simulink model "TST_SATELLITE_A_FAIRE"  (Simulink 8.2)
settings: Solver=ode45  StartTime=0.0  StopTime=60  RelTol=1e-3
values from neighbouring files (symbols this model uses):
  qsc_I_ini = [0 0 0 1]'    [iniSATELLITE.m]
  RW1axe_B = [1 0 0]'    [iniSATELLITE.m]
  RW1inertie_inv = 1/RW1inertie    (= 2439.02439024)    [iniSATELLITE.m]
  RW2axe_B = [0 1 0]'    [iniSATELLITE.m]
  RW2inertie_inv = 1/RW2inertie    (= 2433.09002433)    [iniSATELLITE.m]
  RW3axe_B = [1 0 0]'    [iniSATELLITE.m]
  RW3inertie_inv = 1/RW3inertie    (= 2427.18446602)    [iniSATELLITE.m]
  SCinertie_inv = inv(SCinertie)    [iniSATELLITE.m]
  tor_mag_B = [-2,1,-3]'*1e-03    [runSATELLITE.m]
libraries: dspmtrx3 x2, vrlib x1
settings Model: Creator=delafontaine  LastModifiedBy=Ouss
settings DebuggingCC: FcnCallInpInsideContextMsg=EnableAllAsWarning

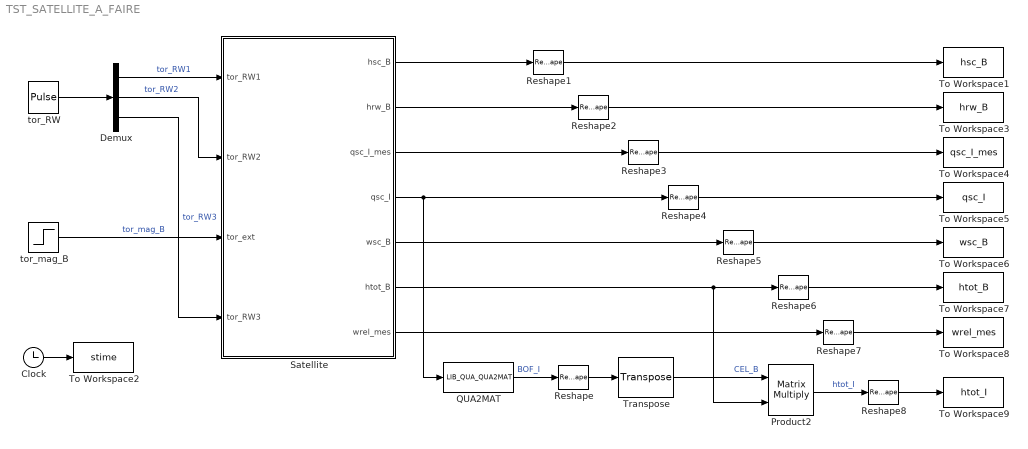
== system TST_SATELLITE_A_FAIRE ==
  Clock : Clock
  Demux : Demux  Outputs=3
  Product2 : Product  Multiplication=Matrix(*)  RndMeth=Zero
  QUA2MAT : MATLABFcn  MATLABFcn=LIB_QUA_QUA2MAT  Output1D=off
  Reshape : Reshape  OutputDimensionality=Customize  OutputDimensions=[3,3]
  Reshape{1..8} (8 alike) : Reshape
  Satellite : Subsystem
  To Workspace1 : ToWorkspace  VariableName=hsc_B  SampleTime=-1
  To Workspace2 : ToWorkspace  VariableName=stime  SampleTime=-1
  To Workspace3 : ToWorkspace  VariableName=hrw_B  SampleTime=-1
  To Workspace4 : ToWorkspace  VariableName=qsc_I_mes  SampleTime=-1
  To Workspace5 : ToWorkspace  VariableName=qsc_I  SampleTime=-1
  To Workspace6 : ToWorkspace  VariableName=wsc_B  SampleTime=-1
  To Workspace7 : ToWorkspace  VariableName=htot_B  SampleTime=-1
  To Workspace8 : ToWorkspace  VariableName=wrel_mes  SampleTime=-1
  To Workspace9 : ToWorkspace  VariableName=htot_I  SampleTime=-1
  "Transpose " : dspmtrx3/Transpose  Hermitian=off  overflowFlag=off
  tor_RW : DiscretePulseGenerator  PulseType=Time based  Amplitude=[0.04, -0.03, 0.05]  Period=[10, 10, 10]  PulseWidth=[20, 30, 40]  PhaseDelay=[2.0, 4.0, 6.0]  VectorParams1D=off
  tor_mag_B : Step  Time=[10, 10, 10]'  Before=[0, 0, 0]'  After=tor_mag_B  SampleTime=0  VectorParams1D=off
  wires:
  Demux/1 -> Satellite/1(tor_RW1)  "tor_RW1"
  Satellite/1(hsc_B) -> Reshape1/1
  Satellite/2(hrw_B) -> Reshape2/1
  Demux/2 -> Satellite/2(tor_RW2)  "tor_RW2"
  Satellite/3(qsc_I_mes) -> Reshape3/1
  tor_mag_B/1 -> Satellite/3(tor_ext)  "tor_mag_B"
  Satellite/4(qsc_I) -> QUA2MAT/1, Reshape4/1
  Satellite/5(wsc_B) -> Reshape5/1
  Satellite/6(htot_B) -> Product2/2, Reshape6/1
  Demux/3 -> Satellite/4(tor_RW3)  "tor_RW3"
  Satellite/7(wrel_mes) -> Reshape7/1
  Clock/1 -> To Workspace2/1
  QUA2MAT/1 -> Reshape/1  "BOF_I"
  "Transpose "/1 -> Product2/1  "CEL_B"
  Product2/1 -> Reshape8/1  "htot_I"
  Reshape/1 -> "Transpose "/1
  tor_RW/1 -> Demux/1
  Reshape1/1 -> To Workspace1/1
  Reshape2/1 -> To Workspace3/1
  Reshape3/1 -> To Workspace4/1
  Reshape4/1 -> To Workspace5/1
  Reshape5/1 -> To Workspace6/1
  Reshape7/1 -> To Workspace8/1
  Reshape8/1 -> To Workspace9/1
  Reshape6/1 -> To Workspace7/1

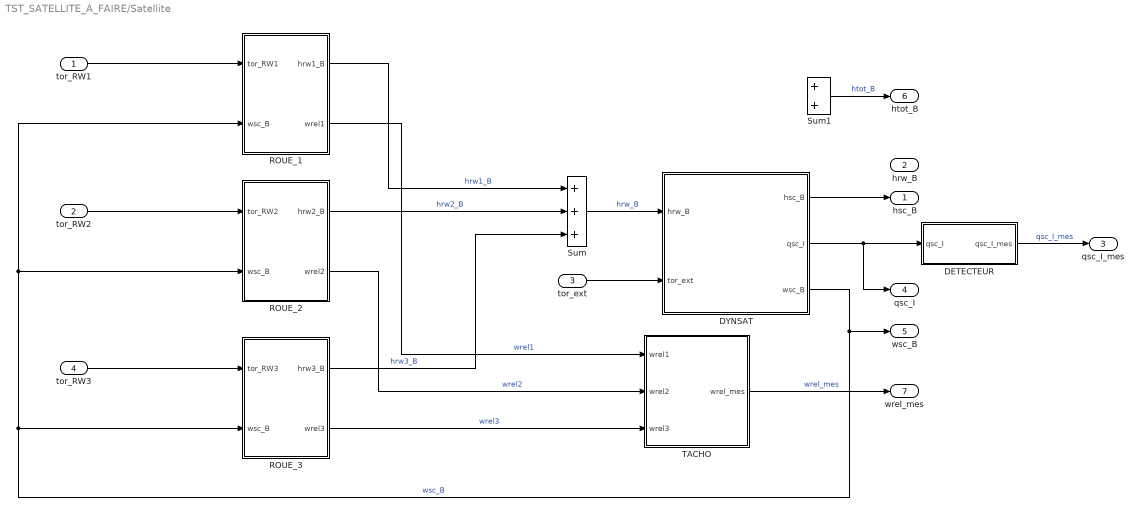
== system TST_SATELLITE_A_FAIRE/Satellite ==
  tor_RW1 : Inport
  tor_RW2 : Inport  Port=2
  tor_ext : Inport  Port=3  PortDimensions=[3,1]
  tor_RW3 : Inport  Port=4
  DETECTEUR : Subsystem
  DYNSAT : Subsystem
  ROUE_1 : Subsystem
  ROUE_2 : Subsystem
  ROUE_3 : Subsystem
  Sum : Sum  Inputs=+++
  Sum1 : Sum
  TACHO : Subsystem
  hsc_B : Outport
  hrw_B : Outport  Port=2
  qsc_I_mes : Outport  Port=3
  qsc_I : Outport  Port=4
  wsc_B : Outport  Port=5
  htot_B : Outport  Port=6
  wrel_mes : Outport  Port=7
  wires:
  DETECTEUR/1(qsc_I_mes) -> qsc_I_mes/1  "qsc_I_mes"
  DYNSAT/2(qsc_I) -> DETECTEUR/1(qsc_I), qsc_I/1
  Sum1/1 -> htot_B/1  "htot_B"
  DYNSAT/1(hsc_B) -> hsc_B/1
  tor_ext/1 -> DYNSAT/2(tor_ext)
  TACHO/1(wrel_mes) -> wrel_mes/1  "wrel_mes"
  Sum/1 -> DYNSAT/1(hrw_B)  "hrw_B"
  DYNSAT/3(wsc_B) -> ROUE_3/2(wsc_B), ROUE_2/2(wsc_B), ROUE_1/2(wsc_B), wsc_B/1  "wsc_B"
  ROUE_3/2(wrel3) -> TACHO/3(wrel3)  "wrel3"
  tor_RW3/1 -> ROUE_3/1(tor_RW3)
  ROUE_3/1(hrw3_B) -> Sum/3  "hrw3_B"
  ROUE_2/2(wrel2) -> TACHO/2(wrel2)  "wrel2"
  tor_RW2/1 -> ROUE_2/1(tor_RW2)
  ROUE_2/1(hrw2_B) -> Sum/2  "hrw2_B"
  ROUE_1/2(wrel1) -> TACHO/1(wrel1)  "wrel1"
  tor_RW1/1 -> ROUE_1/1(tor_RW1)
  ROUE_1/1(hrw1_B) -> Sum/1  "hrw1_B"

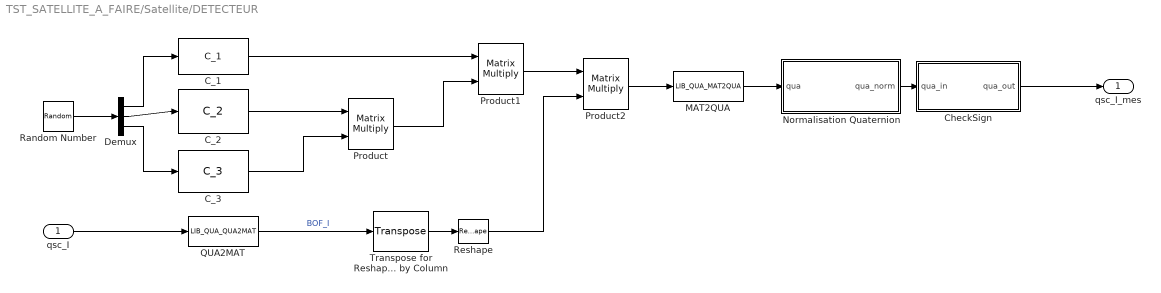
== system TST_SATELLITE_A_FAIRE/Satellite/DETECTEUR ==
  qsc_I : Inport
  C_1 : MATLABFcn  MATLABFcn=C_1  OutputDimensions=[3,3]  Output1D=off
  C_2 : MATLABFcn  MATLABFcn=C_2  OutputDimensions=[3,3]  Output1D=off
  C_3 : MATLABFcn  MATLABFcn=C_3  OutputDimensions=[3,3]  Output1D=off
  CheckSign : MATLAB Function  TreatAsAtomicUnit=on
  Demux : Demux  Outputs=3
  MAT2QUA : MATLABFcn  MATLABFcn=LIB_QUA_MAT2QUA  OutputDimensions=[4,1]  Output1D=off
  Normalisation Quaternion : MATLAB Function  TreatAsAtomicUnit=on
  Product : Product  Multiplication=Matrix(*)  RndMeth=Zero
  Product1 : Product  Multiplication=Matrix(*)  RndMeth=Zero
  Product2 : Product  Multiplication=Matrix(*)  RndMeth=Zero
  QUA2MAT : MATLABFcn  MATLABFcn=LIB_QUA_QUA2MAT
  Random Number : RandomNumber  Mean=[0, 0, 0]  Variance=[1, 1, 1]/1000  Seed=[293343544, 2098503295, 0394802]  SampleTime=0.01  VectorParams1D=off
  Reshape : Reshape  OutputDimensionality=Customize  OutputDimensions=[3,3]
  Transpose for Reshape by Column : dspmtrx3/Transpose  Hermitian=off  overflowFlag=off
  qsc_I_mes : Outport
  wires:
  Random Number/1 -> Demux/1
  Demux/1 -> C_1/1
  Demux/2 -> C_2/1
  Demux/3 -> C_3/1
  C_2/1 -> Product/1
  C_3/1 -> Product/2
  Product/1 -> Product1/2
  C_1/1 -> Product1/1
  QUA2MAT/1 -> Transpose for Reshape by Column/1  "BOF_I"
  Product1/1 -> Product2/1
  Product2/1 -> MAT2QUA/1
  MAT2QUA/1 -> Normalisation Quaternion/1(qua)
  CheckSign/1(qua_out) -> qsc_I_mes/1
  Reshape/1 -> Product2/2
  Transpose for Reshape by Column/1 -> Reshape/1
  qsc_I/1 -> QUA2MAT/1
  Normalisation Quaternion/1(qua_norm) -> CheckSign/1(qua_in)

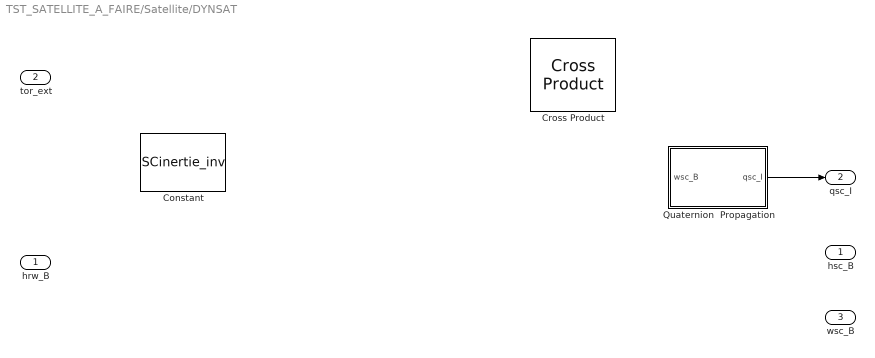
== system TST_SATELLITE_A_FAIRE/Satellite/DYNSAT ==
  hrw_B : Inport
  tor_ext : Inport  Port=2
  Constant : Constant  Value=SCinertie_inv  VectorParams1D=off
  Cross Product : vrlib/Utilities/Cross Product
  Quaternion  Propagation : Subsystem
  hsc_B : Outport
  qsc_I : Outport  Port=2
  wsc_B : Outport  Port=3
  wires:
  Quaternion  Propagation/1(qsc_I) -> qsc_I/1

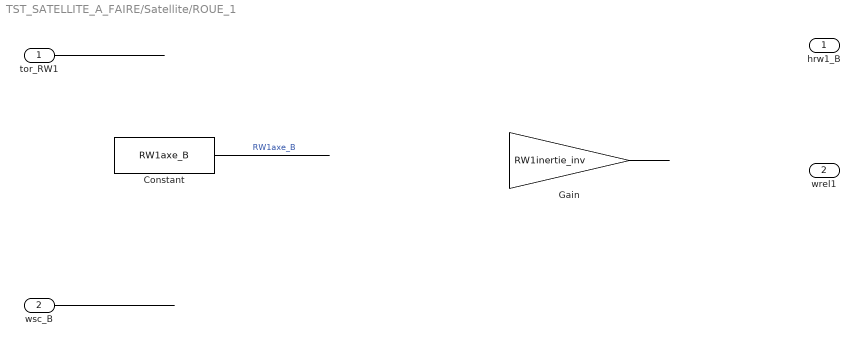
== system TST_SATELLITE_A_FAIRE/Satellite/ROUE_1 ==
  tor_RW1 : Inport
  wsc_B : Inport  Port=2  PortDimensions=[3,1]
  Constant : Constant  Value=RW1axe_B  VectorParams1D=off
  Gain : Gain  Gain=RW1inertie_inv
  hrw1_B : Outport
  wrel1 : Outport  Port=2
  wires:
  tor_RW1/1 -> ?
  Constant/1 -> ?  "RW1axe_B"
  wsc_B/1 -> ?
  Gain/1 -> ?

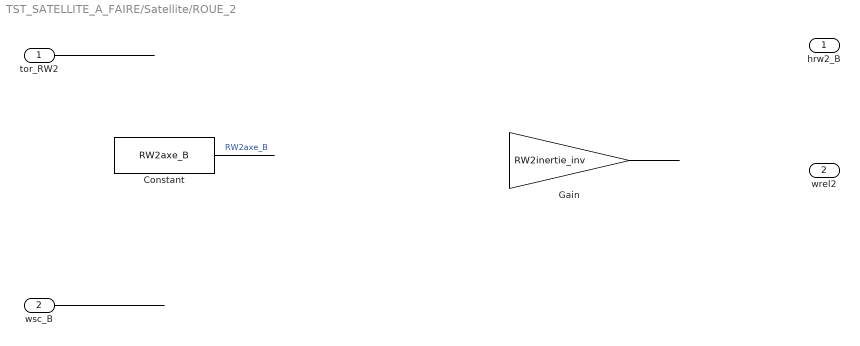
== system TST_SATELLITE_A_FAIRE/Satellite/ROUE_2 ==
  tor_RW2 : Inport
  wsc_B : Inport  Port=2  PortDimensions=[3,1]
  Constant : Constant  Value=RW2axe_B  VectorParams1D=off
  Gain : Gain  Gain=RW2inertie_inv
  hrw2_B : Outport
  wrel2 : Outport  Port=2
  wires:
  Constant/1 -> ?  "RW2axe_B"
  tor_RW2/1 -> ?
  wsc_B/1 -> ?
  Gain/1 -> ?

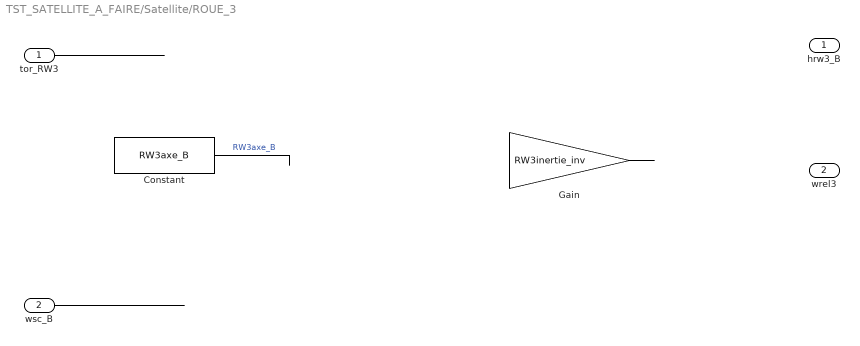
== system TST_SATELLITE_A_FAIRE/Satellite/ROUE_3 ==
  tor_RW3 : Inport
  wsc_B : Inport  Port=2  PortDimensions=[3,1]
  Constant : Constant  Value=RW3axe_B  VectorParams1D=off
  Gain : Gain  Gain=RW3inertie_inv
  hrw3_B : Outport
  wrel3 : Outport  Port=2
  wires:
  tor_RW3/1 -> ?
  wsc_B/1 -> ?
  Constant/1 -> ?  "RW3axe_B"
  Gain/1 -> ?

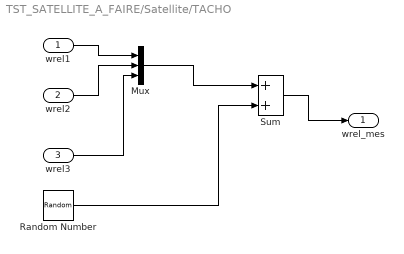
== system TST_SATELLITE_A_FAIRE/Satellite/TACHO ==
  wrel1 : Inport
  wrel2 : Inport  Port=2
  wrel3 : Inport  Port=3
  Mux : Mux  Inputs=3
  Random Number : RandomNumber  Mean=[0, 0, 0]  Variance=[1, 1, 1]  Seed=[293343544, 2098503295, 0394802]  SampleTime=0.1
  Sum : Sum
  wrel_mes : Outport
  wires:
  wrel1/1 -> Mux/1
  wrel2/1 -> Mux/2
  wrel3/1 -> Mux/3
  Mux/1 -> Sum/1
  Random Number/1 -> Sum/2
  Sum/1 -> wrel_mes/1

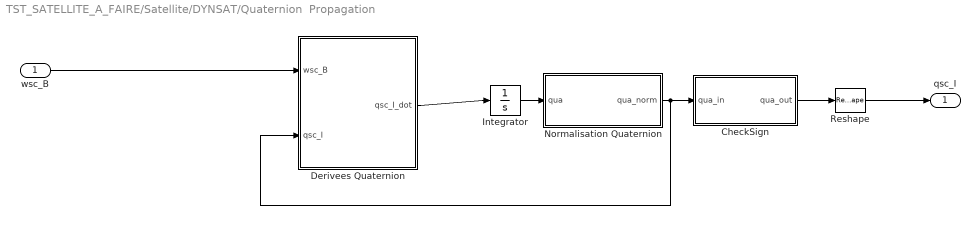
== system TST_SATELLITE_A_FAIRE/Satellite/DYNSAT/Quaternion  Propagation ==
  wsc_B : Inport
  CheckSign : MATLAB Function  TreatAsAtomicUnit=on
  Derivees Quaternion : MATLAB Function  TreatAsAtomicUnit=on
  Integrator : Integrator  InitialCondition=qsc_I_ini
  Normalisation Quaternion : MATLAB Function  TreatAsAtomicUnit=on
  Reshape : Reshape  OutputDimensionality=Column vector (2-D)
  qsc_I : Outport
  wires:
  wsc_B/1 -> Derivees Quaternion/1(wsc_B)
  Derivees Quaternion/1(qsc_I_dot) -> Integrator/1
  Integrator/1 -> Normalisation Quaternion/1(qua)
  Normalisation Quaternion/1(qua_norm) -> Derivees Quaternion/2(qsc_I), CheckSign/1(qua_in)
  CheckSign/1(qua_out) -> Reshape/1
  Reshape/1 -> qsc_I/1

== matlab function Satellite/DYNSAT/Quaternion Propagation/Normalisation Quaternion ==
  data: qua input double; qua_norm output double
  function qua_norm = normalisation(qua)
% #codegen

  qua_norm = zeros(4,1);
  
  temp = qua(1)*qua(1) + qua(2)*qua(2) + qua(3)*qua(3) + qua(4)*qua(4);

  if temp <= 0.0 
     for i=1:3
        qua_norm(i) = 0.0;
     end;
     qua_norm(4) = 1.0;
  else
     temp = sqrt(temp);
     for i=1:4
        qua_norm(i) = qua(i)/temp;
     end;
  end

== matlab function Satellite/DYNSAT/Quaternion Propagation/Derivees Quaternion ==
  data: wsc_B input double; qsc_I_dot output double; qsc_I input double
function qsc_I_dot = quaternion_propag(wsc_B, qsc_I)
%#codegen

  qsc_I_dot = zeros(4,1);
  
  qsc_I_dot(1,1) = 0.5*( wsc_B(3,1)*qsc_I(2,1)-wsc_B(2,1)*qsc_I(3,1)+wsc_B(1,1)*qsc_I(4,1));
  qsc_I_dot(2,1) = 0.5*(-wsc_B(3,1)*qsc_I(1,1)+wsc_B(1,1)*qsc_I(3,1)+wsc_B(2,1)*qsc_I(4,1));
  qsc_I_dot(3,1) = 0.5*( wsc_B(2,1)*qsc_I(1,1)-wsc_B(1,1)*qsc_I(2,1)+wsc_B(3,1)*qsc_I(4,1));
  qsc_I_dot(4,1) = 0.5*(-wsc_B(1,1)*qsc_I(1,1)-wsc_B(2,1)*qsc_I(2,1)-wsc_B(3,1)*qsc_I(3,1));

== matlab function Satellite/DYNSAT/Quaternion Propagation/CheckSign ==
  data: qua_in input double; qua_out output double
  function qua_out = checksign(qua_in)
% #codegen

  qua_out = zeros(4,1);

  if qua_in(4) < 0.0 
      qua_out = -qua_in;
  else
      qua_out = qua_in;
  end

== matlab function Satellite/DETECTEUR/CheckSign ==
  data: qua_in input double; qua_out output double
  function qua_out = checksign(qua_in)
% #codegen

  qua_out = zeros(4,1);

  if qua_in(4) < 0.0 
      qua_out = -qua_in;
  else
      qua_out = qua_in;
  end

== matlab function Satellite/DETECTEUR/Normalisation Quaternion ==
  data: qua input double; qua_norm output double
  function qua_norm = normalisation(qua)
% #codegen

  qua_norm = zeros(4,1);
  
  temp = qua(1)*qua(1) + qua(2)*qua(2) + qua(3)*qua(3) + qua(4)*qua(4);

  if temp <= 0.0 
     for i=1:3
        qua_norm(i) = 0.0;
     end;
     qua_norm(4) = 1.0;
  else
     temp = sqrt(temp);
     for i=1:4
        qua_norm(i) = qua(i)/temp;
     end;
  end
